simulink model "s_function"  (R2021a)
settings: Solver=VariableStepAuto  StartTime=0.0  StopTime=10.0  RelTol=1e-3
libraries: simulink x2
settings Model: Creator=Sai229  LastModifiedBy=Sai229

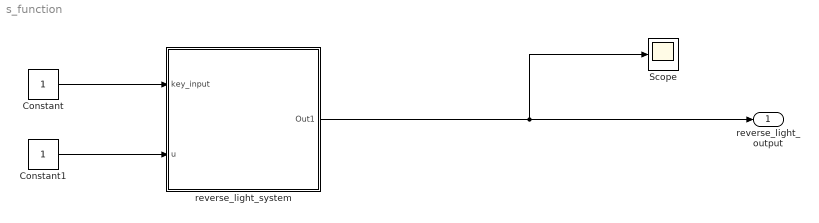
== system s_function ==
  Constant : Constant
  Constant1 : Constant
  Scope : Scope
  reverse_light_system : Subsystem  TreatAsAtomicUnit=on  mask{Parameter1=0, time_period=0.1}
      mask prompts: time_period "Enter the time period for blinking the light"
  reverse_light_output : Outport
  wires:
  reverse_light_system/1(Out1) -> Scope/1, reverse_light_output/1
  Constant/1 -> reverse_light_system/1(key_input)
  Constant1/1 -> reverse_light_system/2(u)

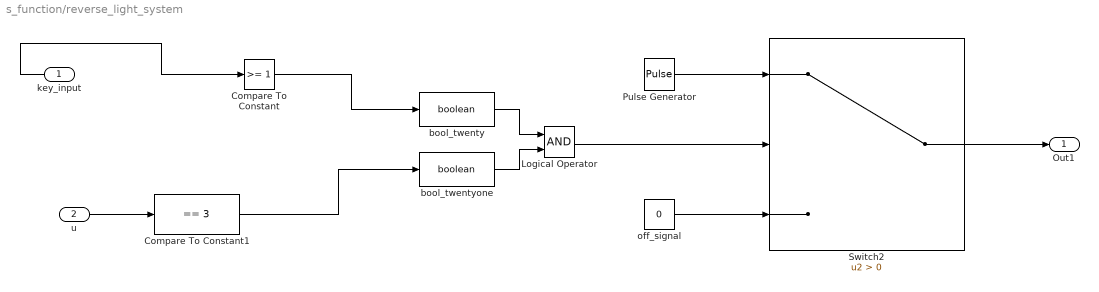
== system s_function/reverse_light_system ==
  key_input : Inport
  u : Inport  Port=2
  Compare To Constant : simulink/Logic and Bit Operations/Compare To Constant  relop=>=  const=1  OutDataTypeStr=boolean
  Compare To Constant1 : simulink/Logic and Bit Operations/Compare To Constant  relop===  const=3  OutDataTypeStr=boolean
  Logical Operator : Logic  AllPortsSameDT=off  OutDataTypeStr=boolean
  Pulse Generator : DiscretePulseGenerator  PulseType=Time based  Amplitude=5  Period=time_period  PulseWidth=50
  Switch2 : Switch  Criteria=u2 > Threshold
  bool_twenty : DataTypeConversion  OutDataTypeStr=boolean
  bool_twentyone : DataTypeConversion  OutDataTypeStr=boolean
  off_signal : Constant  Value=0
  Out1 : Outport
  wires:
  Switch2/1 -> Out1/1
  Logical Operator/1 -> Switch2/2
  bool_twentyone/1 -> Logical Operator/2
  off_signal/1 -> Switch2/3
  Pulse Generator/1 -> Switch2/1
  bool_twenty/1 -> Logical Operator/1
  key_input/1 -> Compare To Constant/1
  Compare To Constant/1 -> bool_twenty/1
  Compare To Constant1/1 -> bool_twentyone/1
  u/1 -> Compare To Constant1/1
